simulink model "omnibundle_control"  (R2018b)
settings: Solver=ode23t  StartTime=0.0  StopTime=20  RelTol=1e-3
values from neighbouring files (symbols this model uses):
  ddqv = ddt(ddt(qv,dts),dts)    [main.m]    (also in traj_planning.m)
  dq0 = [0 0 0]'    [main.m]
  dqv = ddt(qv,dts)    [main.m]    (also in traj_planning.m)
  Km = inv(fv)    [main.m]
  Kp = wn^2./diag(Km)./Kv    [main.m]
  Kv = 2*zeta*wn./diag(Km)    [main.m]
  q0 = qs(1,2:4)'    [main.m]
  qv = []    [main.m]    (also in traj_planning.m)
  tau_d = [0;0.1;0]    [main.m]
  Tv = diag(Tm)    [main.m]
undefined symbols (not defined in the file or in its folder): ddpev, dpev, pev, te, tq
libraries: simulink x12, quarc_library x4
settings Model: Creator=lucas  LastModifiedBy=lucas
settings SolverCC: ZeroCrossAlgorithm=Adaptive
settings DebuggingCC: IgnoredZcDiagnostic=none

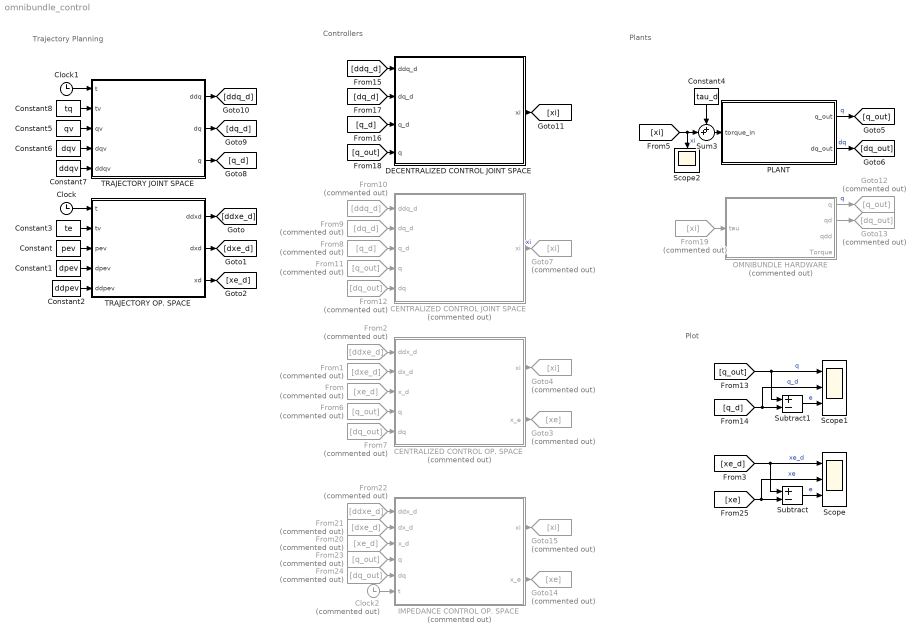
== system omnibundle_control ==
  note: Plot
  note: Plants
  note: Controllers
  note: Trajectory Planning
  CENTRALIZED CONTROL JOINT SPACE : MATLAB Function  Commented=on  TreatAsAtomicUnit=on
  CENTRALIZED CONTROL OP. SPACE : MATLAB Function  Commented=on  TreatAsAtomicUnit=on
  Clock : Clock
  Clock1 : Clock
  Clock2 : Clock  Commented=on
  Constant : Constant  Value=pev
  Constant1 : Constant  Value=dpev
  Constant2 : Constant  Value=ddpev
  Constant3 : Constant  Value=te
  Constant4 : Constant  Value=tau_d
  Constant5 : Constant  Value=qv
  Constant6 : Constant  Value=dqv
  Constant7 : Constant  Value=ddqv
  Constant8 : Constant  Value=tq
  DECENTRALIZED CONTROL JOINT SPACE : Subsystem
  From : From  Commented=on  GotoTag=xe_d
  From1 : From  Commented=on  GotoTag=dxe_d
  From10 : From  Commented=on  GotoTag=ddq_d
  From11 : From  Commented=on  GotoTag=q_out
  From12 : From  Commented=on  GotoTag=dq_out
  From19 : From  Commented=on  GotoTag=xi
  From2 : From  Commented=on  GotoTag=ddxe_d
  From20 : From  Commented=on  GotoTag=xe_d
  From21 : From  Commented=on  GotoTag=dxe_d
  From22 : From  Commented=on  GotoTag=ddxe_d
  From23 : From  Commented=on  GotoTag=q_out
  From24 : From  Commented=on  GotoTag=dq_out
  From6 : From  Commented=on  GotoTag=q_out
  From7 : From  Commented=on  GotoTag=dq_out
  From8 : From  Commented=on  GotoTag=q_d
  From9 : From  Commented=on  GotoTag=dq_d
  Goto12 : Goto  Commented=on  GotoTag=q_out
  Goto13 : Goto  Commented=on  GotoTag=dq_out
  Goto14 : Goto  Commented=on  GotoTag=xe
  Goto15 : Goto  Commented=on  GotoTag=xi
  Goto3 : Goto  Commented=on  GotoTag=xe
  Goto4 : Goto  Commented=on  GotoTag=xi
  Goto7 : Goto  Commented=on  GotoTag=xi
  IMPEDANCE CONTROL OP. SPACE : MATLAB Function  Commented=on  TreatAsAtomicUnit=on
  OMNIBUNDLE HARDWARE : Subsystem  Commented=on
      mask DialogControl DescGroupVar Prompt: Omni
      mask DialogControl DescTextVar Prompt: This block contains a simple controller for the omni haptic device.
  PLANT : Subsystem
  Scope : Scope  NumInputPorts=3
  Scope1 : Scope  NumInputPorts=3
  Scope2 : Scope
  Subtract : Sum  Inputs=+-
  Subtract1 : Sum  Inputs=+-
  Sum3 : Sum  Inputs=++|
  TRAJECTORY JOINT SPACE : MATLAB Function  TreatAsAtomicUnit=on
  TRAJECTORY OP. SPACE : MATLAB Function  TreatAsAtomicUnit=on
  wires:
  From/1 -> CENTRALIZED CONTROL OP. SPACE/3(x_d)
  Clock/1 -> TRAJECTORY OP. SPACE/1(t)
  PLANT/1(q_out) -> [q_out]  "q"
  From2/1 -> CENTRALIZED CONTROL OP. SPACE/1(ddx_d)
  From1/1 -> CENTRALIZED CONTROL OP. SPACE/2(dx_d)
  CENTRALIZED CONTROL OP. SPACE/1(xi) -> Goto4/1
  Constant1/1 -> TRAJECTORY OP. SPACE/4(dpev)
  Constant2/1 -> TRAJECTORY OP. SPACE/5(ddpev)
  Constant/1 -> TRAJECTORY OP. SPACE/3(pev)
  Constant3/1 -> TRAJECTORY OP. SPACE/2(tv)
  Sum3/1 -> PLANT/1(torque_in)
  Constant4/1 -> Sum3/1
  Subtract/1 -> Scope/3  "e"
  PLANT/2(dq_out) -> [dq_out]  "dq"
  TRAJECTORY OP. SPACE/1(ddxd) -> [ddxe_d]
  TRAJECTORY OP. SPACE/2(dxd) -> [dxe_d]
  TRAJECTORY OP. SPACE/3(xd) -> [xe_d]
  [xe_d] -> Subtract/1, Scope/1  "xe_d"
  CENTRALIZED CONTROL OP. SPACE/2(x_e) -> Goto3/1
  [xe] -> Scope/2, Subtract/2  "xe"
  [xi] -> Scope2/1, Sum3/2  "xi"
  From6/1 -> CENTRALIZED CONTROL OP. SPACE/4(q)
  From7/1 -> CENTRALIZED CONTROL OP. SPACE/5(dq)
  Subtract1/1 -> Scope1/3  "e"
  Constant8/1 -> TRAJECTORY JOINT SPACE/2(tv)
  Clock1/1 -> TRAJECTORY JOINT SPACE/1(t)
  Constant7/1 -> TRAJECTORY JOINT SPACE/5(ddqv)
  Constant6/1 -> TRAJECTORY JOINT SPACE/4(dqv)
  Constant5/1 -> TRAJECTORY JOINT SPACE/3(qv)
  CENTRALIZED CONTROL JOINT SPACE/1(xi) -> Goto7/1  "xi"
  TRAJECTORY JOINT SPACE/3(q) -> [q_d]
  TRAJECTORY JOINT SPACE/2(dq) -> [dq_d]
  TRAJECTORY JOINT SPACE/1(ddq) -> [ddq_d]
  From9/1 -> CENTRALIZED CONTROL JOINT SPACE/2(dq_d)
  From8/1 -> CENTRALIZED CONTROL JOINT SPACE/3(q_d)
  From10/1 -> CENTRALIZED CONTROL JOINT SPACE/1(ddq_d)
  From11/1 -> CENTRALIZED CONTROL JOINT SPACE/4(q)
  From12/1 -> CENTRALIZED CONTROL JOINT SPACE/5(dq)
  [q_out] -> Subtract1/1, Scope1/1  "q"
  [q_d] -> Scope1/2, Subtract1/2  "q_d"
  DECENTRALIZED CONTROL JOINT SPACE/1(xi) -> [xi]
  [ddq_d] -> DECENTRALIZED CONTROL JOINT SPACE/1(ddq_d)
  [q_d] -> DECENTRALIZED CONTROL JOINT SPACE/3(q_d)
  [dq_d] -> DECENTRALIZED CONTROL JOINT SPACE/2(dq_d)
  [q_out] -> DECENTRALIZED CONTROL JOINT SPACE/4(q)
  From19/1 -> OMNIBUNDLE HARDWARE/1(tau)
  OMNIBUNDLE HARDWARE/1(q) -> Goto12/1  "q"
  OMNIBUNDLE HARDWARE/2(qd) -> Goto13/1
  IMPEDANCE CONTROL OP. SPACE/1(xi) -> Goto15/1
  From24/1 -> IMPEDANCE CONTROL OP. SPACE/5(dq)
  From21/1 -> IMPEDANCE CONTROL OP. SPACE/2(dx_d)
  From23/1 -> IMPEDANCE CONTROL OP. SPACE/4(q)
  IMPEDANCE CONTROL OP. SPACE/2(x_e) -> Goto14/1
  From20/1 -> IMPEDANCE CONTROL OP. SPACE/3(x_d)
  From22/1 -> IMPEDANCE CONTROL OP. SPACE/1(ddx_d)
  Clock2/1 -> IMPEDANCE CONTROL OP. SPACE/6(t)

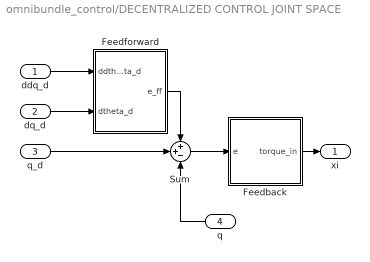
== system omnibundle_control/DECENTRALIZED CONTROL JOINT SPACE ==
  ddq_d : Inport
  dq_d : Inport  Port=2
  q_d : Inport  Port=3
  q : Inport  Port=4
  Feedback : Subsystem
  Feedforward : Subsystem
  Sum : Sum  Inputs=++-
  xi : Outport
  wires:
  ddq_d/1 -> Feedforward/1(ddtheta_d)
  q_d/1 -> Sum/2
  Feedforward/1(e_ff) -> Sum/1
  Sum/1 -> Feedback/1(e)
  Feedback/1(torque_in) -> xi/1
  q/1 -> Sum/3
  dq_d/1 -> Feedforward/2(dtheta_d)

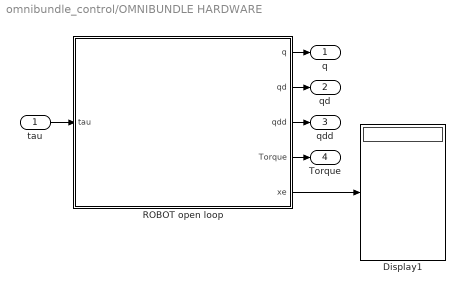
== system omnibundle_control/OMNIBUNDLE HARDWARE ==
  tau : Inport
  Display1 : Display
  ROBOT open loop : Subsystem
  q : Outport
  qd : Outport  Port=2
  qdd : Outport  Port=3
  Torque : Outport  Port=4
  wires:
  ROBOT open loop/1(q) -> q/1
  ROBOT open loop/2(qd) -> qd/1
  ROBOT open loop/3(qdd) -> qdd/1
  ROBOT open loop/4(Torque) -> Torque/1
  ROBOT open loop/5(xe) -> Display1/1
  tau/1 -> ROBOT open loop/1(tau)

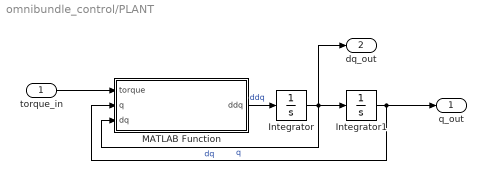
== system omnibundle_control/PLANT ==
  torque_in : Inport
  Integrator : Integrator  InitialCondition=dq0
  Integrator1 : Integrator  InitialCondition=q0
  MATLAB Function : MATLAB Function  TreatAsAtomicUnit=on
  q_out : Outport
  dq_out : Outport  Port=2
  wires:
  MATLAB Function/1(ddq) -> Integrator/1  "ddq"
  Integrator/1 -> dq_out/1, MATLAB Function/3(dq), Integrator1/1  "dq"
  Integrator1/1 -> q_out/1, MATLAB Function/2(q)  "q"
  torque_in/1 -> MATLAB Function/1(torque)

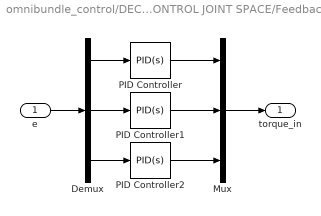
== system omnibundle_control/DECENTRALIZED CONTROL JOINT SPACE/Feedback ==
  e : Inport
  Demux : Demux  Outputs=3
  Mux : Mux  Inputs=3
  PID Controller : simulink/Continuous/PID Controller  Controller=PID  Form=Parallel  TimeDomain=Continuous-time  SampleTime=-1  IntegratorMethod=Forward Euler  FilterMethod=Forward Euler  ControllerParametersSource=internal  P=Kv(1)+Kp(1)*Kv(1)*Tv(1)  I=Kp(1)*Kv(1)  D=Kv(1)*Tv(1)  UseFilter=on  N=1000  TunerSelectOption=Transfer Function Based (PID Tuner App)  ZeroCross=off  InitialConditionSource=internal  InitialConditionForIntegrator=0  InitialConditionForFilter=0  DifferentiatorICPrevScaledInput=0  ExternalReset=none  TrackingMode=off  Kt=1  LimitOutput=off  UpperSaturationLimit=inf  LowerSaturationLimit=-inf  LinearizeAsGain=on  AntiWindupMode=none  Kb=1  POutMin=[]  POutMax=[]  IOutMin=[]  IOutMax=[]  DOutMin=[]  DOutMax=[]  NOutMin=[]  NOutMax=[]  SumOutMin=[]  SumOutMax=[]  SaturationOutMin=[]  SaturationOutMax=[]  PParamMin=[]  PParamMax=[]  IParamMin=[]  IParamMax=[]  DParamMin=[]  DParamMax=[]  NParamMin=[]  NParamMax=[]  KbParamMin=[]  KbParamMax=[]  KtParamMin=[]  KtParamMax=[]  KbOutMin=[]  KbOutMax=[]  KtOutMin=[]  KtOutMax=[]  IntegratorOutMin=[]  IntegratorOutMax=[]  FilterOutMin=[]  FilterOutMax=[]  SumI1OutMin=[]  SumI1OutMax=[]  SumI2OutMin=[]  SumI2OutMax=[]  SumI3OutMin=[]  SumI3OutMax=[]  SumI4OutMin=[]  SumI4OutMax=[]  SumDOutMin=[]  SumDOutMax=[]  DifferentiatorOutMin=[]  DifferentiatorOutMax=[]  FilterDiffOutCoefMin=[]  FilterDiffOutCoefMax=[]  ReciprocalOutMin=[]  ReciprocalOutMax=[]  SumDenOutMin=[]  SumDenOutMax=[]  SumNumOutMin=[]  SumNumOutMax=[]  DivideOutMin=[]  DivideOutMax=[]  IntegratorContinuousStateAttributes=''  IntegratorStateMustResolveToSignalObject=off  IntegratorRTWStateStorageClass=Auto  FilterContinuousStateAttributes=''  FilterStateMustResolveToSignalObject=off  FilterRTWStateStorageClass=Auto  ParallelPVariant=InternalParameters  IdealPVariant=Disabled  IVariant=InternalParameters  DVariant=InternalParameters  IntegratorVariant=Continuous  SatVariant=Disabled  AWVariant=Passthrough  PCopyVariant=Disabled  TRVariant=Disabled  FdbkBlocksVariant=Forward  IdealPFdbkVariant=Disabled  SatFdbkVariant=Disabled  DerivativeFilterVariant=ContFilter  NVariant=InternalParameters  NCopyVariant=Disabled  FilterICVariant=InternalICsFilter  IntegratorICVariant=InternalICs  ExternalResetVariant=Disabled  TRSumVariant=Passthrough  SumFdbkVariant=Disabled  SumVariant=Sum_PID
  PID Controller1 : simulink/Continuous/PID Controller  Controller=PID  Form=Parallel  TimeDomain=Continuous-time  SampleTime=-1  IntegratorMethod=Forward Euler  FilterMethod=Forward Euler  ControllerParametersSource=internal  P=Kv(2)+Kp(2)*Kv(2)*Tv(2)  I=Kp(2)*Kv(2)  D=Kv(2)*Tv(2)  UseFilter=on  N=1000  TunerSelectOption=Transfer Function Based (PID Tuner App)  ZeroCross=off  InitialConditionSource=internal  InitialConditionForIntegrator=0  InitialConditionForFilter=0  DifferentiatorICPrevScaledInput=0  ExternalReset=none  TrackingMode=off  Kt=1  LimitOutput=off  UpperSaturationLimit=inf  LowerSaturationLimit=-inf  LinearizeAsGain=on  AntiWindupMode=none  Kb=1  POutMin=[]  POutMax=[]  IOutMin=[]  IOutMax=[]  DOutMin=[]  DOutMax=[]  NOutMin=[]  NOutMax=[]  SumOutMin=[]  SumOutMax=[]  SaturationOutMin=[]  SaturationOutMax=[]  PParamMin=[]  PParamMax=[]  IParamMin=[]  IParamMax=[]  DParamMin=[]  DParamMax=[]  NParamMin=[]  NParamMax=[]  KbParamMin=[]  KbParamMax=[]  KtParamMin=[]  KtParamMax=[]  KbOutMin=[]  KbOutMax=[]  KtOutMin=[]  KtOutMax=[]  IntegratorOutMin=[]  IntegratorOutMax=[]  FilterOutMin=[]  FilterOutMax=[]  SumI1OutMin=[]  SumI1OutMax=[]  SumI2OutMin=[]  SumI2OutMax=[]  SumI3OutMin=[]  SumI3OutMax=[]  SumI4OutMin=[]  SumI4OutMax=[]  SumDOutMin=[]  SumDOutMax=[]  DifferentiatorOutMin=[]  DifferentiatorOutMax=[]  FilterDiffOutCoefMin=[]  FilterDiffOutCoefMax=[]  ReciprocalOutMin=[]  ReciprocalOutMax=[]  SumDenOutMin=[]  SumDenOutMax=[]  SumNumOutMin=[]  SumNumOutMax=[]  DivideOutMin=[]  DivideOutMax=[]  IntegratorContinuousStateAttributes=''  IntegratorStateMustResolveToSignalObject=off  IntegratorRTWStateStorageClass=Auto  FilterContinuousStateAttributes=''  FilterStateMustResolveToSignalObject=off  FilterRTWStateStorageClass=Auto  ParallelPVariant=InternalParameters  IdealPVariant=Disabled  IVariant=InternalParameters  DVariant=InternalParameters  IntegratorVariant=Continuous  SatVariant=Disabled  AWVariant=Passthrough  PCopyVariant=Disabled  TRVariant=Disabled  FdbkBlocksVariant=Forward  IdealPFdbkVariant=Disabled  SatFdbkVariant=Disabled  DerivativeFilterVariant=ContFilter  NVariant=InternalParameters  NCopyVariant=Disabled  FilterICVariant=InternalICsFilter  IntegratorICVariant=InternalICs  ExternalResetVariant=Disabled  TRSumVariant=Passthrough  SumFdbkVariant=Disabled  SumVariant=Sum_PID
  PID Controller2 : simulink/Continuous/PID Controller  Controller=PID  Form=Parallel  TimeDomain=Continuous-time  SampleTime=-1  IntegratorMethod=Forward Euler  FilterMethod=Forward Euler  ControllerParametersSource=internal  P=Kv(3)+Kp(3)*Kv(3)*Tv(3)  I=Kp(3)*Kv(3)  D=Kv(3)*Tv(3)  UseFilter=on  N=1000  TunerSelectOption=Transfer Function Based (PID Tuner App)  ZeroCross=off  InitialConditionSource=internal  InitialConditionForIntegrator=0  InitialConditionForFilter=0  DifferentiatorICPrevScaledInput=0  ExternalReset=none  TrackingMode=off  Kt=1  LimitOutput=off  UpperSaturationLimit=inf  LowerSaturationLimit=-inf  LinearizeAsGain=on  AntiWindupMode=none  Kb=1  POutMin=[]  POutMax=[]  IOutMin=[]  IOutMax=[]  DOutMin=[]  DOutMax=[]  NOutMin=[]  NOutMax=[]  SumOutMin=[]  SumOutMax=[]  SaturationOutMin=[]  SaturationOutMax=[]  PParamMin=[]  PParamMax=[]  IParamMin=[]  IParamMax=[]  DParamMin=[]  DParamMax=[]  NParamMin=[]  NParamMax=[]  KbParamMin=[]  KbParamMax=[]  KtParamMin=[]  KtParamMax=[]  KbOutMin=[]  KbOutMax=[]  KtOutMin=[]  KtOutMax=[]  IntegratorOutMin=[]  IntegratorOutMax=[]  FilterOutMin=[]  FilterOutMax=[]  SumI1OutMin=[]  SumI1OutMax=[]  SumI2OutMin=[]  SumI2OutMax=[]  SumI3OutMin=[]  SumI3OutMax=[]  SumI4OutMin=[]  SumI4OutMax=[]  SumDOutMin=[]  SumDOutMax=[]  DifferentiatorOutMin=[]  DifferentiatorOutMax=[]  FilterDiffOutCoefMin=[]  FilterDiffOutCoefMax=[]  ReciprocalOutMin=[]  ReciprocalOutMax=[]  SumDenOutMin=[]  SumDenOutMax=[]  SumNumOutMin=[]  SumNumOutMax=[]  DivideOutMin=[]  DivideOutMax=[]  IntegratorContinuousStateAttributes=''  IntegratorStateMustResolveToSignalObject=off  IntegratorRTWStateStorageClass=Auto  FilterContinuousStateAttributes=''  FilterStateMustResolveToSignalObject=off  FilterRTWStateStorageClass=Auto  ParallelPVariant=InternalParameters  IdealPVariant=Disabled  IVariant=InternalParameters  DVariant=InternalParameters  IntegratorVariant=Continuous  SatVariant=Disabled  AWVariant=Passthrough  PCopyVariant=Disabled  TRVariant=Disabled  FdbkBlocksVariant=Forward  IdealPFdbkVariant=Disabled  SatFdbkVariant=Disabled  DerivativeFilterVariant=ContFilter  NVariant=InternalParameters  NCopyVariant=Disabled  FilterICVariant=InternalICsFilter  IntegratorICVariant=InternalICs  ExternalResetVariant=Disabled  TRSumVariant=Passthrough  SumFdbkVariant=Disabled  SumVariant=Sum_PID
  torque_in : Outport
  wires:
  Mux/1 -> torque_in/1
  e/1 -> Demux/1
  Demux/1 -> PID Controller/1
  PID Controller/1 -> Mux/1
  Demux/3 -> PID Controller2/1
  PID Controller2/1 -> Mux/3
  Demux/2 -> PID Controller1/1
  PID Controller1/1 -> Mux/2

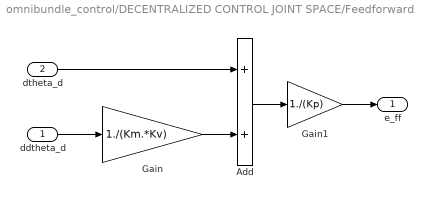
== system omnibundle_control/DECENTRALIZED CONTROL JOINT SPACE/Feedforward ==
  ddtheta_d : Inport
  dtheta_d : Inport  Port=2
  Add : Sum
  Gain : Gain  Gain=1./(Km.*Kv)
  Gain1 : Gain  Gain=1./(Kp)
  e_ff : Outport
  wires:
  Add/1 -> Gain1/1
  dtheta_d/1 -> Add/1
  ddtheta_d/1 -> Gain/1
  Gain/1 -> Add/2
  Gain1/1 -> e_ff/1

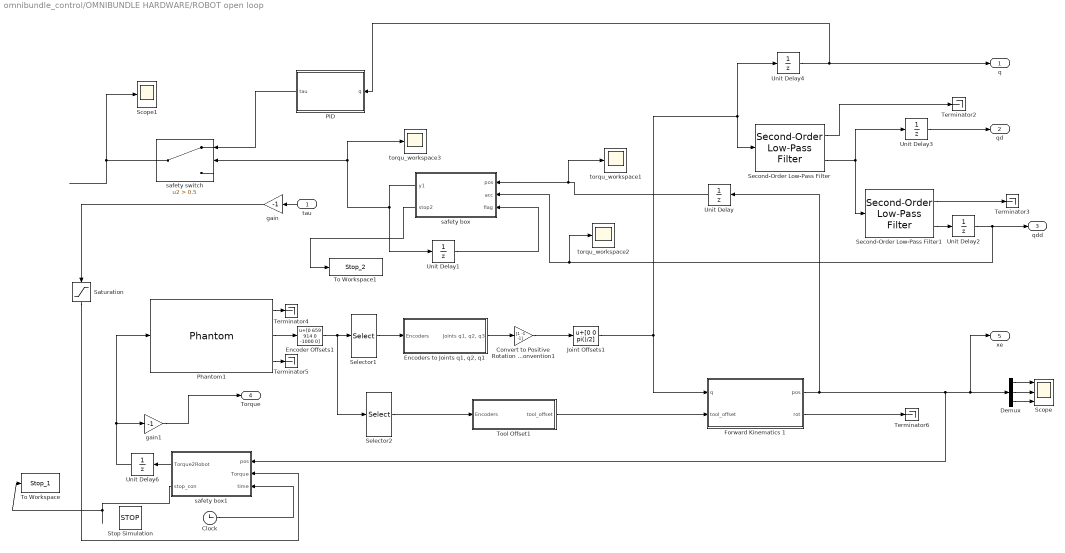
== system omnibundle_control/OMNIBUNDLE HARDWARE/ROBOT open loop ==
  tau : Inport
  Clock : Clock
  Convert to Positive Rotation Convention1 : Gain  Gain=[1 -1 -1]
  Demux : Demux  Outputs=3
  Encoder Offsets1 : Bias  Bias=[0 659 914 0 -1000 0]
  "Encoders to Joints q1, q2, q1" : Subsystem
  Forward Kinematics 1 : MATLAB Function  TreatAsAtomicUnit=on
  Joint Offsets1 : Bias  Bias=[0 0 pi()/2]
  PID : Subsystem
  Phantom1 : quarc_library/Devices/Third-Party/SensAble/Phantom/Phantom  device_name=Default Device  output_type=Encoders Values  input_type=Joint space  velocity_limit_option=on  velocity_limit=1200  is_7dof=off  sample_time=-1
      settings: AttributesFormatString=(%<device_name>)
  Saturation : Saturate  UpperLimit=0.3  LowerLimit=-0.3
  Scope : Scope  NumInputPorts=3
  Scope1 : Scope
  Second-Order Low-Pass Filter : quarc_library/Continuous/Second-Order Low-Pass Filter  params_source=Internal (dialog parameters)  input_width=10  input_zeta=1  input_init=0
  Second-Order Low-Pass Filter1 : quarc_library/Continuous/Second-Order Low-Pass Filter  params_source=Internal (dialog parameters)  input_width=10  input_zeta=1  input_init=0
  Selector1 : Selector  InputPortWidth=6  IndexOptions=Index vector (dialog)  Indices=[1:3]  OutputSizes=1
  Selector2 : Selector  InputPortWidth=6  IndexOptions=Index vector (dialog)  Indices=[4:6]  OutputSizes=1
  Stop Simulation : Stop
  Terminator{2..6} (5 alike) : Terminator
  To Workspace : ToWorkspace  VariableName=Stop_1  SampleTime=-1
  To Workspace1 : ToWorkspace  VariableName=Stop_2  SampleTime=-1
  Tool Offset1 : MATLAB Function  TreatAsAtomicUnit=on
  Unit Delay : UnitDelay  InitialCondition=[0.1 0 0]'  SampleTime=-1
  Unit Delay{1..4,6} (5 alike) : UnitDelay  SampleTime=-1
  gain : Gain  Gain=-1
  gain1 : Gain  Gain=-1
  safety box : MATLAB Function  TreatAsAtomicUnit=on
  safety box1 : MATLAB Function  TreatAsAtomicUnit=on
  safety switch : Switch  Criteria=u2 > Threshold  Threshold=0.5  SampleTime=1e-3
  torqu_workspace1 : Scope
  torqu_workspace2 : Scope
  torqu_workspace3 : Scope
  q : Outport
  qd : Outport  Port=2
  qdd : Outport  Port=3
  Torque : Outport  Port=4
  xe : Outport  Port=5
  wires:
  Second-Order Low-Pass Filter/1 -> Terminator2/1
  Second-Order Low-Pass Filter1/1 -> Terminator3/1
  Second-Order Low-Pass Filter/2 -> Unit Delay3/1, Second-Order Low-Pass Filter1/1
  Convert to Positive Rotation Convention1/1 -> Joint Offsets1/1
  Phantom1/2 -> Encoder Offsets1/1
  Phantom1/3 -> Terminator5/1
  Phantom1/1 -> Terminator4/1
  Selector1/1 -> "Encoders to Joints q1, q2, q1"/1(Encoders)
  Encoder Offsets1/1 -> Selector2/1, Selector1/1
  "Encoders to Joints q1, q2, q1"/1("Joints q1, q2, q3") -> Convert to Positive Rotation Convention1/1
  Joint Offsets1/1 -> Unit Delay4/1, Second-Order Low-Pass Filter/1, Forward Kinematics 1/1(q)
  Forward Kinematics 1/2(rot) -> Terminator6/1
  Selector2/1 -> Tool Offset1/1(Encoders)
  Tool Offset1/1(tool_offset) -> Forward Kinematics 1/2(tool_offset)
  Demux/1 -> Scope/1
  Demux/2 -> Scope/2
  Demux/3 -> Scope/3
  tau/1 -> gain/1
  gain/1 -> Saturation/1
  safety box/1(y1) -> torqu_workspace3/1, safety switch/2, Unit Delay1/1
  safety switch/1 -> Scope1/1
  Unit Delay/1 -> torqu_workspace1/1, safety box/1(pos)
  Unit Delay1/1 -> safety box/3(flag)
  Second-Order Low-Pass Filter1/2 -> Unit Delay2/1
  Unit Delay2/1 -> torqu_workspace2/1, safety box/2(acc), qdd/1
  Unit Delay3/1 -> qd/1
  Unit Delay4/1 -> PID/1(q), q/1
  PID/1(tau) -> safety switch/1
  Clock/1 -> safety box1/3(time)
  safety box1/1(Torque2Robot) -> Unit Delay6/1
  safety box1/2(stop_con) -> To Workspace/1
  Forward Kinematics 1/1(pos) -> Unit Delay/1, safety box1/1(pos), xe/1, Demux/1
  Unit Delay6/1 -> Phantom1/1, gain1/1
  gain1/1 -> Torque/1
  Saturation/1 -> safety box1/2(Torque)
  safety box/2(stop2) -> To Workspace1/1

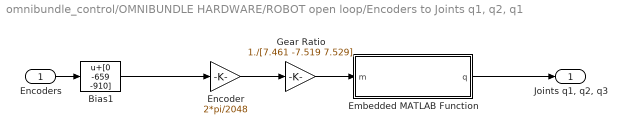
== system omnibundle_control/OMNIBUNDLE HARDWARE/ROBOT open loop/Encoders to Joints q1, q2, q1 ==
  Encoders : Inport
  Bias1 : Bias  Bias=[0 -659 -910]
  Embedded MATLAB Function : MATLAB Function  TreatAsAtomicUnit=on
  Encoder : Gain  Gain=2*pi/2048
  Gear Ratio : Gain  Gain=1./[7.461 -7.519 7.529]
  "Joints q1, q2, q3" : Outport
  wires:
  Embedded MATLAB Function/1(q) -> "Joints q1, q2, q3"/1
  Encoders/1 -> Bias1/1
  Encoder/1 -> Gear Ratio/1
  Gear Ratio/1 -> Embedded MATLAB Function/1(m)
  Bias1/1 -> Encoder/1

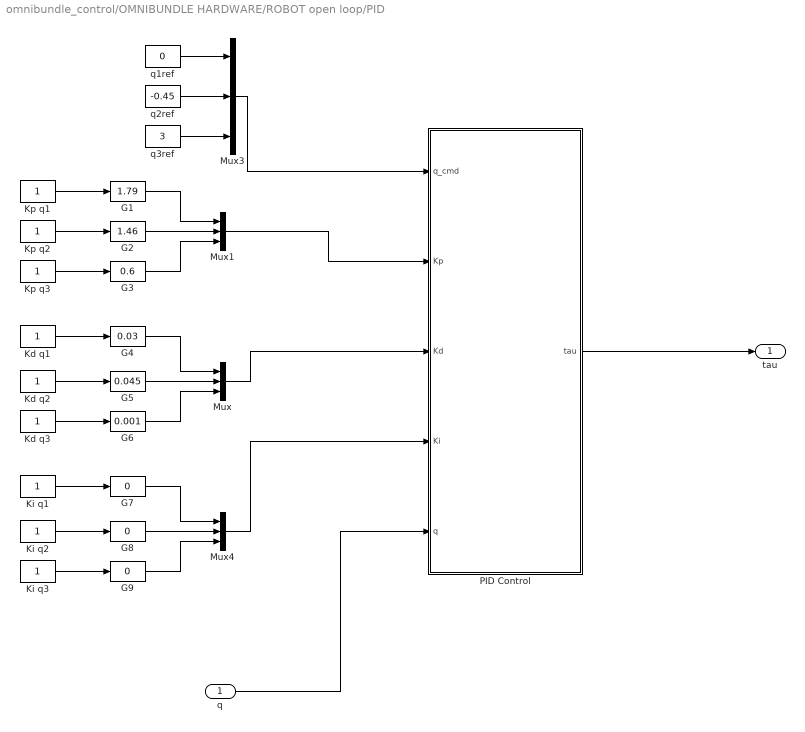
== system omnibundle_control/OMNIBUNDLE HARDWARE/ROBOT open loop/PID ==
  q : Inport
  G1 : simulink/Math Operations/Slider Gain  gain=1.79  low=0  high=2
  G2 : simulink/Math Operations/Slider Gain  gain=1.46  low=0  high=2
  G3 : simulink/Math Operations/Slider Gain  gain=0.6  low=0  high=1
  G4 : simulink/Math Operations/Slider Gain  gain=0.03  low=0.02  high=0.1
  G5 : simulink/Math Operations/Slider Gain  gain=0.045  low=0.02  high=0.1
  G6 : simulink/Math Operations/Slider Gain  gain=0.001  low=0  high=0.025
  G7 : simulink/Math Operations/Slider Gain  gain=0  low=0  high=2
  G8 : simulink/Math Operations/Slider Gain  gain=0  low=0  high=2
  G9 : simulink/Math Operations/Slider Gain  gain=0  low=0  high=3
  Kd q1 : Constant
  Kd q2 : Constant
  Kd q3 : Constant
  Ki q1 : Constant
  Ki q2 : Constant
  Ki q3 : Constant
  Kp q1 : Constant
  Kp q2 : Constant
  Kp q3 : Constant
  Mux{,1,3..4} (4 alike) : Mux  Inputs=3
  PID Control : Subsystem
  q1ref : Constant  Value=0
  q2ref : Constant  Value=-0.45
  q3ref : Constant  Value=3
  tau : Outport
  wires:
  Mux3/1 -> PID Control/1(q_cmd)
  Mux/1 -> PID Control/3(Kd)
  Mux1/1 -> PID Control/2(Kp)
  Kp q1/1 -> G1/1
  Kp q2/1 -> G2/1
  Kp q3/1 -> G3/1
  Kd q1/1 -> G4/1
  Kd q2/1 -> G5/1
  Kd q3/1 -> G6/1
  G1/1 -> Mux1/1
  G2/1 -> Mux1/2
  G3/1 -> Mux1/3
  G4/1 -> Mux/1
  G5/1 -> Mux/2
  G6/1 -> Mux/3
  Ki q1/1 -> G7/1
  Ki q2/1 -> G8/1
  Ki q3/1 -> G9/1
  G7/1 -> Mux4/1
  G8/1 -> Mux4/2
  G9/1 -> Mux4/3
  Mux4/1 -> PID Control/4(Ki)
  PID Control/1(tau) -> tau/1
  q/1 -> PID Control/5(q)
  q1ref/1 -> Mux3/1
  q2ref/1 -> Mux3/2
  q3ref/1 -> Mux3/3

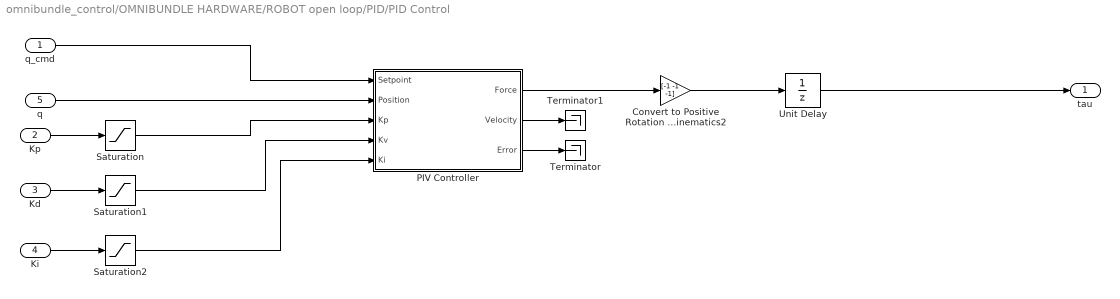
== system omnibundle_control/OMNIBUNDLE HARDWARE/ROBOT open loop/PID/PID Control ==
  q_cmd : Inport
  Kp : Inport  Port=2
  Kd : Inport  Port=3
  Ki : Inport  Port=4
  q : Inport  Port=5
  Convert to Positive Rotation Convension Used in Kinematics2 : Gain  Gain=[-1 -1 -1]
  PIV Controller : Subsystem
  Saturation : Saturate  UpperLimit=[2 2 1]  LowerLimit=[0 0 0]
  Saturation1 : Saturate  UpperLimit=[.1 .1 .025]  LowerLimit=[.02 .02 0]
  Saturation2 : Saturate  UpperLimit=[2 2 3]  LowerLimit=[0 0 0]
  Terminator : Terminator
  Terminator1 : Terminator
  Unit Delay : UnitDelay  SampleTime=-1
  tau : Outport
  wires:
  Saturation2/1 -> PIV Controller/5(Ki)
  Ki/1 -> Saturation2/1
  Saturation1/1 -> PIV Controller/4(Kv)
  Kd/1 -> Saturation1/1
  Saturation/1 -> PIV Controller/3(Kp)
  Kp/1 -> Saturation/1
  q_cmd/1 -> PIV Controller/1(Setpoint)
  PIV Controller/2(Velocity) -> Terminator1/1
  PIV Controller/3(Error) -> Terminator/1
  PIV Controller/1(Force) -> Convert to Positive Rotation Convension Used in Kinematics2/1
  Convert to Positive Rotation Convension Used in Kinematics2/1 -> Unit Delay/1
  Unit Delay/1 -> tau/1
  q/1 -> PIV Controller/2(Position)

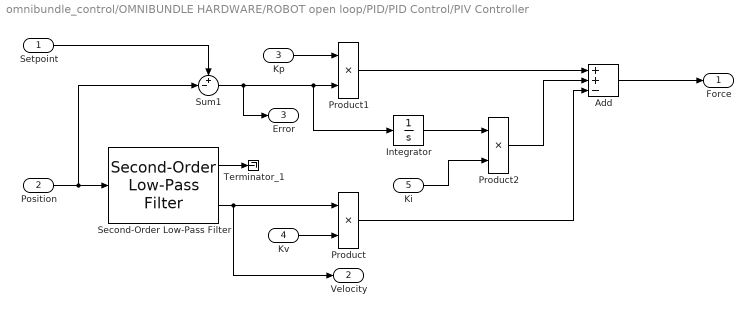
== system omnibundle_control/OMNIBUNDLE HARDWARE/ROBOT open loop/PID/PID Control/PIV Controller ==
  Setpoint : Inport
  Position : Inport  Port=2
  Kp : Inport  Port=3
  Kv : Inport  Port=4
  Ki : Inport  Port=5
  Add : Sum  Inputs=++-
  Integrator : Integrator
  Product : Product  RndMeth=Zero
  Product1 : Product  RndMeth=Zero
  Product2 : Product  RndMeth=Zero
  Second-Order Low-Pass Filter : quarc_library/Continuous/Second-Order Low-Pass Filter  params_source=Internal (dialog parameters)  input_width=200  input_zeta=1  input_init=0
  Sum1 : Sum  Inputs=+-|
  Terminator_1 : Terminator
  Force : Outport
  Velocity : Outport  Port=2
  Error : Outport  Port=3
  wires:
  Position/1 -> Sum1/2, Second-Order Low-Pass Filter/1
  Second-Order Low-Pass Filter/2 -> Velocity/1, Product/1
  Kp/1 -> Product1/1
  Setpoint/1 -> Sum1/1
  Sum1/1 -> Error/1, Product1/2, Integrator/1
  Kv/1 -> Product/2
  Second-Order Low-Pass Filter/1 -> Terminator_1/1
  Integrator/1 -> Product2/1
  Ki/1 -> Product2/2
  Product1/1 -> Add/1
  Product2/1 -> Add/2
  Product/1 -> Add/3
  Add/1 -> Force/1

== matlab function omnibundle_control/OMNIBUNDLE HARDWARE/ROBOT open loop/Encoders to Joints q1, q2, q1/Embedded MATLAB Function ==
  data: m input; q output
function q = Motors_2_Joints(m)
q = m;
q(1) = m(1);
q(2) = m(2);
q(3) = m(3) - m(2) -pi/2;
end

== matlab function omnibundle_control/PLANT/MATLAB Function ==
  data: torque input; q input; dq input; ddq output
function ddq = omnibundle_dyn(torque,q,dq)
    
    ddq = dyn_omni_bundle_fun(9.8, q, dq, torque);

== matlab function omnibundle_control/TRAJECTORY OP. SPACE ==
  data: t input; tv input; ddxd output; dxd output; xd output; pev input; dpev input; ddpev input
function [ddxd,dxd,xd] = trajectory_planning(t, tv, pev, dpev, ddpev)

    xd   = zeros(3,1);
    dxd  = zeros(3,1);
    ddxd = zeros(3,1);

    if t > tv(end-2)
        t = tv(end-2);
    end

    xd = interp1(tv',pev',t)';
    dxd = interp1(tv(1:end-1)',dpev',t)';
    ddxd = interp1(tv(1:end-2)',ddpev',t)';

== matlab function omnibundle_control/TRAJECTORY JOINT SPACE ==
  data: t input; tv input; ddq output; dq output; q output; qv input; dqv input; ddqv input
function [ddq,dq,q] = trajectory_planning(t, tv, qv, dqv, ddqv)

    if t > tv(end-2)
        t = tv(end-2);
    end

    q = interp1(tv',qv',t)';
    dq = interp1(tv(1:end-1)',dqv',t)';
    ddq = interp1(tv(1:end-2)',ddqv',t)';

== matlab function omnibundle_control/OMNIBUNDLE HARDWARE/ROBOT open loop/Forward Kinematics 1 ==
  data: pos output; q input; rot output; tool_offset input
function [pos,rot]    = ForwardKinematics(q,tool_offset)
% This block supports the Embedded MATLAB subset.
% See the help menu for details. 

% Link lengths
L1 = .132;
L2 = .132;

%Define A-matrices
%A1= DH(theta ,d ,a ,alpha)
A1 = DH(q(1), 0, 0, -pi()/2);
A2 = DH(q(2), 0, L1, 0);
A3 = DH(q(3)-pi/2, 0, L2, 0);

%Define T Matrices
T01=A1;
T02=T01*A2;
T03=T02*A3;

%tool_offset given with respect to frame 3.
T_tool=T03*tool_offset;
rot=T_tool(1:3,1:3);
pos=T_tool(1:3,4);

%Axes of rotation in base coordinates. 
z0=[0 0 1]';
z1=T01(1:3,3);
z2=T02(1:3,3);

%Coordinate Frame origins in Base frame coordinates
p0=[0 0 0]';
p1=T01(1:3,4);
p2=T02(1:3,4);
p3=T03(1:3,4);

%Formulation of the Jacobian

%%%%%%%%%%%%%%%%%%%%%%%%%%%%%%%%%%%%%%%%%%%%%%%%%%%%
%jac = [cross(z0,(pos-p0)) cross(z1,(pos-p1)) cross(z2,(pos-p2))
 %   z0 z1 z2];

end

function A = DH(theta, d, a, alpha)

A_R_z = [cos(theta) -sin(theta) 0 0;
         sin(theta) cos(theta) 0 0;
         0 0 1 0;
         0 0 0 1];

A_T_z = [1 0 0 0;
         0 1 0 0;
         0 0 1 d;
         0 0 0 1];
     
  

A_T_x = [1 0 0 a;
         0 1 0 0;
         0 0 1 0;
         0 0 0 1];

A_R_x = [1 0 0 0;
         0 cos(alpha) -sin(alpha)  0;
         0 sin(alpha) cos(alpha) 0;
         0 0 0 1];

A = A_R_z*A_T_z*A_T_x*A_R_x;

end

== matlab function omnibundle_control/CENTRALIZED CONTROL JOINT SPACE ==
  data: ddq_d input; dq_d input; q_d input; q input; dq input; xi output
function xi = centr_control_joint_space(ddq_d, dq_d, q_d, q, dq)

    % initialize output
    xi = zeros(3,1);

    % controller gains
    zeta = 1;
    wn = 20;
    K_D = diag(repmat(2*zeta*wn,3,1));
    K_P = diag(repmat(wn^2,3,1));
    
    % desired joint acceleration
    y = ddq_d + K_P * ( q_d - q ) + K_D * ( dq_d - dq );

    % inverse dynamics
    xi = inv_dyn_omni_bundle_fun(9.8, q, dq, y);

== matlab function omnibundle_control/OMNIBUNDLE HARDWARE/ROBOT open loop/safety box1 ==
  data: pos input; Torque input; Torque2Robot output; time input; stop_con output
function [Torque2Robot,stop_con] = fcn(pos,Torque,time)

% gives 0 input torque if x,y,z are out of the safety box or the max
% acceleration is exceeded
stop_con=0;

x=pos(1);
y=pos(2);
z=pos(3);

xmin = 0.16-0.01;
xmax = 0.16+0.01;
ymin = 0-0.01;
ymax = 0+0.01;
zmin = -0.13-0.01;
zmax = -0.13+0.01;

if (time<0.002)
    if x<xmin || x>xmax || y<ymin || y>ymax || z<zmin || z>zmax
        stop_con=1;
    end
end

Torque2Robot = Torque;

== matlab function omnibundle_control/CENTRALIZED CONTROL OP. SPACE ==
  data: ddx_d input; dx_d input; x_d input; q input; dq input; xi output; x_e output
function [xi, x_e] = control_centr_operspace(ddx_d, dx_d, x_d, q, dq)

    % initialize output
    xi = zeros(3,1);

    % direct dynamics
    x_e = dir_kin_omni_bundle_fun(q);
    
    % direct differential kinematics
    A_0_e = A_0_e_omni_bundle_fun(q);
    eulZYZ = rotm2eul(A_0_e(1:3,1:3),'ZYZ')';
    J_A = anal_jacob_omni_bundle_fun(q,eulZYZ);
    dx_e = J_A(1:3,1:3) * dq;
    
    % dJA*dq
    dJ_A = dJ_analit_P_omni_bundle_fun(q,dq);
    
    % controller gains
    zeta = 1;
    wn = 20;
    K_D = diag(repmat(2*zeta*wn,3,1));
    K_P = diag(repmat(wn^2,3,1));
    
    % desired end-effector acceleration
    z = ddx_d + K_P * (x_d - x_e) + K_D * (dx_d - dx_e);
    
    % inverse differential kinematics - desired joints acceleration
    y = J_A(1:3,1:3) \ ( z - dJ_A * dq ); % 
    
    % inverse dynamics
    xi = inv_dyn_omni_bundle_fun(9.8, q, dq, y);

== matlab function omnibundle_control/OMNIBUNDLE HARDWARE/ROBOT open loop/Tool Offset1 ==
  data: Encoders input; tool_offset output
function tool_offset = getToolOffset(Encoders)

%convert encoder values to angles using bias and gain
bias = [-2048 -2654 -2048];
gain = [2*pi()/4915 2*pi()/4096 2*pi()/4915];
Angle = (Encoders' + bias).*gain;

% convert the angle to the positive rotation convention defined
% by DH parameters
pos_rot = [-1 1 1];
joint_offset = [0 -(40-180)*pi/180 0];
Joint456 = Angle.*pos_rot + joint_offset;

%pick off theta4 and theta5
theta4 = Joint456(1);
theta5 = Joint456(2);

% The orientation of the tool offset matrix is given two successive
% rotations about x and z axis. 
RotZ = [cos(theta5) -sin(theta5) 0; sin(theta5) cos(theta5) 0; 0 0 1];
RotX = [1 0 0; 0 cos(theta4) -sin(theta4); 0 sin(theta4) cos(theta4)];
R = RotX*RotZ; % R is the rotation matrix of the tool offset matrix with respect to frame 3

% with respect to frame 3, the tool is 0.039m in the x-direction. Convert
% this vector to tool frame coordinates
tool_pos =R * [.039; 0; 0];

%create a Tool_offset transformation matrix. Use Identity matrix for
%rotation to show that the end effector frame and frame 3 are always
%aligned
I = [1 0 0; 0 1 0; 0 0 1];
tool = cat(2,I,tool_pos);
tool_offset = cat(1,tool,[0 0 0 1]);

== matlab function omnibundle_control/OMNIBUNDLE HARDWARE/ROBOT open loop/safety box ==
  data: pos input; acc input; y1 output; flag input; stop2 output
function [y1,stop2] = fcn(pos,acc,flag)

% gives 0 input torque if x,y,z are out of the safety box or the max
% acceleration is exceeded

stop2 = 0;

x=pos(1);
y=pos(2);
z=pos(3);

% xmin = -0.22;
% xmax = 0.22;
% ymin = -0.1;
% ymax = 0.1;
% zmin = -0.14;
% zmax = 0.04;
xmin = 0.1;
xmax = 0.3;
ymin = -0.1;
ymax = 0.1;
zmin = -0.14;
zmax = 0.05;

acc1 = abs(acc(1));
acc2 = abs(acc(2));
acc3 = abs(acc(3));
acc_max = [30; 30; 60];

if flag==0
    if x<xmin || x>xmax || y<ymin || y>ymax || z<zmin || z>zmax || acc1>acc_max(1) || acc2>acc_max(2) || acc3>acc_max(3)
        flag=1;
        stop2 = 1;
    end
end

y1 = flag;

== matlab function omnibundle_control/IMPEDANCE CONTROL OP. SPACE ==
  data: ddx_d input; dx_d input; x_d input; q input; dq input; xi output; x_e output; t input
function [xi, x_e] = control_impedance_operspace(ddx_d, dx_d, x_d, q, dq, t)

    % initialize output
    xi = zeros(3,1);

    % direct dynamics
    x_e = dir_kin_omni_bundle_fun(q);
    
    % direct differential kinematics
    A_0_e = A_0_e_omni_bundle_fun(q);
    eulZYZ = rotm2eul(A_0_e(1:3,1:3),'ZYZ')';
    J_A = anal_jacob_omni_bundle_fun(q,eulZYZ);
    dx_e = J_A(1:3,1:3) * dq;
    
    % dJA*dq
    dJ_A = dJ_analit_P_omni_bundle_fun(q,dq);
    
    % controller gains
    zeta = 2;
    wn = 10;
    
%     zeta = 0.5;
%     wn = 10; 
    
    M_D = 0.01*eye(3);
    K_D = M_D * diag(repmat(2*zeta*wn,3,1));
    K_P = M_D * diag(repmat(wn^2,3,1));
    
    
    % desired end-effector acceleration
    z = M_D \ ( M_D * ddx_d + K_P * (x_d - x_e) + K_D * (dx_d - dx_e) );
     
    % inverse differential dynamics - desired joints acceleration
    y = J_A(1:3,1:3) \ ( z - dJ_A * dq ); % 
    
    % inverse dynamics
    xi = inv_dyn_omni_bundle_fun(9.8, q, dq, y);
    
    
    if t>=10
        xi = xi + J_A(1:3,1:3)*[1 0 0]';     % apply disturbance in x direction
    end
